simulink model "step_11"  (R2014b)
settings: Solver=ode45  StartTime=0.0  StopTime=10.0  RelTol=1e-3
values from neighbouring files (symbols this model uses):
  A = sys.a    [MinSeg_Parameters.m]    (also in MinSeg_Parameters_v2.m = [0, 1, 0, 0; Arow12, Arow22, 0, Arow24; 0, 0, 0, 1; Arow41, ; MinSeg_Parameters_v3.m = [0, 1, 0, 0; Arow12, Arow22, 0, Arow24; 0, 0, 0, 1; Arow41, )
  B = sys.b    [MinSeg_Parameters.m]    (also in MinSeg_Parameters_v2.m = [0; Brow2; 0; Brow3]; MinSeg_Parameters_v3.m = [0; Brow2; 0; Brow3])
  C = sys.c    [MinSeg_Parameters.m]    (also in MinSeg_Parameters_v2.m = eye(N); MinSeg_Parameters_v3.m = eye(N))
  D = sys.d    [MinSeg_Parameters.m]    (also in MinSeg_Parameters_v2.m = zeros(N, 1); MinSeg_Parameters_v3.m = zeros(N, 1))
  L = 0.11    [MinSeg_Parameters.m]
undefined symbols (not defined in the file or in its folder): xhatini, xini
settings Model: Creator=mo114c  LastModifiedBy=mo114c
settings DebuggingCC: UnderspecifiedInitializationDetection=Classic  MergeDetectMultiDrivingBlocksExec=none  SolverPrmCheckMsg=none  StateNameClashWarn=warning

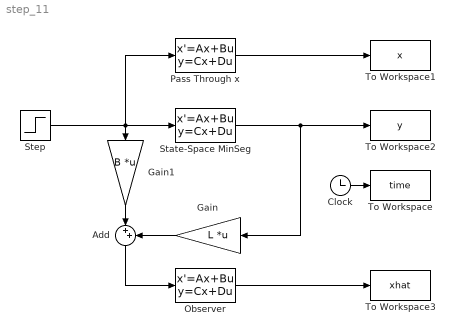
== system step_11 ==
  Add : Sum  Inputs=|++
  Clock : Clock
  Gain : Gain  Gain=L  Multiplication=Matrix(K*u)
  Gain1 : Gain  Gain=B  Multiplication=Matrix(K*u)
  Observer : StateSpace  A=A-L*C  B=eye(size(A))  C=eye(size(A))  D=zeros(size(A))  X0=xhatini
  Pass Through x : StateSpace  A=A  B=B  C=eye(size(A))  D=zeros(size(C,1),size(B,2))  X0=xini
  State-Space MinSeg : StateSpace  A=A  B=B  C=C  D=D  X0=xini
  Step : Step  SampleTime=0
  To Workspace : ToWorkspace  VariableName=time  SampleTime=-1
  To Workspace1 : ToWorkspace  VariableName=x  SampleTime=-1
  To Workspace2 : ToWorkspace  VariableName=y  SampleTime=-1
  To Workspace3 : ToWorkspace  VariableName=xhat  SampleTime=-1
  wires:
  Clock/1 -> To Workspace/1
  Step/1 -> Pass Through x/1, Gain1/1, State-Space MinSeg/1
  Pass Through x/1 -> To Workspace1/1
  State-Space MinSeg/1 -> To Workspace2/1, Gain/1
  Gain/1 -> Add/2
  Gain1/1 -> Add/1
  Add/1 -> Observer/1
  Observer/1 -> To Workspace3/1
